simulink model "PMT_MPPT"  (Simulink 8.4)
settings: Solver=ode45  StartTime=0.0  StopTime=8  FixedStep=2.5e-6  RelTol=1e-3
undefined symbols (not defined in the file): Cin, Cout, Cp, G, Isc, L1a, L1b, Rload, Rload1, Rload2, sigbuilder_block, T1, T2, Temp, Tsampling, Voc
libraries: powerlib x19, simulink x3, powerlib_extras x1, fuzblock x1
settings Model: Creator=daoxuanb  LastModifiedBy=Administrator

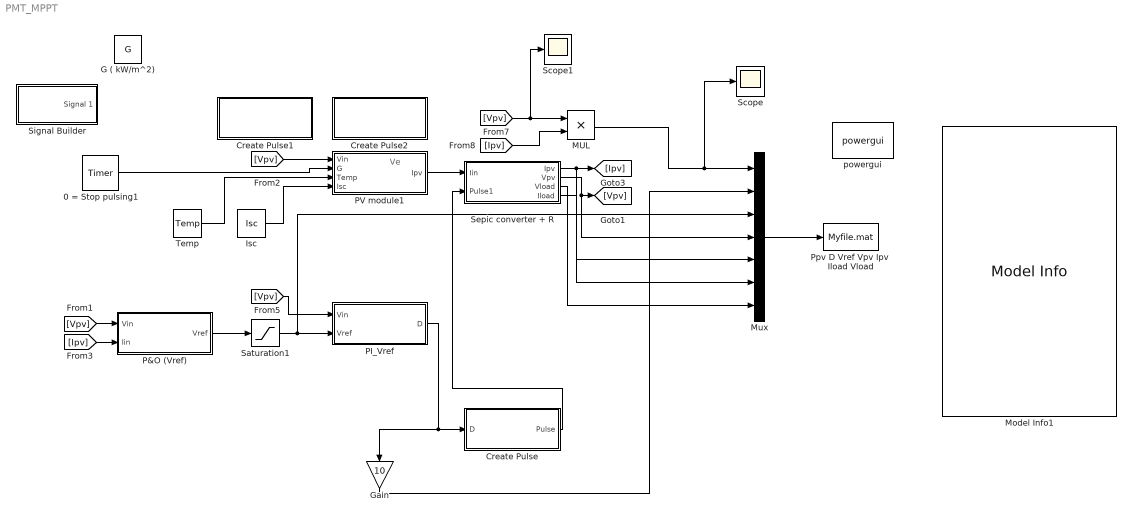
== system PMT_MPPT ==
  note: Ve
  0 = Stop pulsing1 : powerlib_extras/Control  Blocks/Timer  t=[0 2 4 6 8 ]  e=[1 0.9 0.8 0.6 0.5 ]
  Create Pulse : Subsystem
  Create Pulse1 : Subsystem
      settings: OpenFcn=thongso1
      mask Display: disp('initiate')
  Create Pulse2 : Subsystem
      settings: OpenFcn=ve1
      mask Display: disp('initiate')
  G ( kW/m^2) : Constant  Value=G
  Gain : Gain  Gain=10
  Isc : Constant  Value=Isc
  MUL : Product  Inputs=**
  Model Info1 : simulink/Model-Wide Utilities/Model Info  BlockCM=None  Frame=on  DisplayStringWithTags=|  HorizontalTextAlignment=Center  LeftAlignmentValue=0.5  SourceBlockDiagram=PMT_MPPT  TagMaxNumber=20
      | PARAMETER:
      | Boost + R:
      | C1 = 1000uF
      | C2 = 1000uF
      | C3 = 1000uF
      | L1 = 222uH
      | L2 = 222uH
      | R   = 20
      | Boost + Motor:
      | C1 = 2200u
      | C2 = 100u
      | L   = 10m
      | R   = 20
      | PI:  P = 0.05  I = 1
      | Pulse: 20000Hz
      | Pmax =  85W
      | Vmpp = 18.18 V
      | Impp   =  4.88 A
      | Voc = 21.85 V
      | Isc = 5.13 A
  Mux : Mux  Inputs=7
  P&O (Vref) : Subsystem
  PI_Vref : Subsystem
  PV module1 : Subsystem
  Ppv D Vref Vpv Ipv  Iload Vload : ToFile  Filename=Myfile.mat  MatrixName=XX
  Saturation1 : Saturate  UpperLimit=21.85  LowerLimit=0
  Scope : Scope
      settings: YMin=30  YMax=90  SaveName=Ppv
  Scope1 : Scope
      settings: YMin=10  YMax=90  SaveName=Ppv1
  Sepic converter + R : Subsystem
  Signal Builder : Subsystem  Tag=STV Subsys  LoadFcn=sigbuilder_block('load');  StartFcn=sigbuilder_block('start');  StopFcn=sigbuilder_block('stop');  ClipboardFcn=sigbuilder_block('clipboard');  mask(Sigbuilder block){}
      mask help: Simulink:masks:SigbuilderBlock_MD
      mask init:
      | if ~strcmp(get_param(bdroot(gcbh),'SimulationStatus'),'stopped') tuvar = sigbuilder_block('maskInit'); end
      settings: CopyFcn=sigbuilder_block('copy');  DeleteFcn=sigbuilder_block('delete');  ModelCloseFcn=sigbuilder_block('modelClose');  PreSaveFcn=sigbuilder_block('preSave');  PauseFcn=sigbuilder_block('pause');  ContinueFcn=sigbuilder_block('continue');  NameChangeFcn=sigbuilder_block('namechange');  OpenFcn=sigbuilder_block('open',[584.25 105.75 550.5 399.75 ]);  CloseFcn=sigbuilder_block('close');
      mask Display: plot(0, 0, 100, 100,[2, 2, 32, 32, 2], [68, 8, 8, 68, 68],[32, 2], [38, 38], [32, 19, 2],[53, 60, 44], [32, 17, 17, 2],[16, 16, 31, 31]);txt = getActiveGroup(gcbh);text(2, 100, txt,'verticalAlignment', 'top');
  "Temp " : Constant  Value=Temp
  powergui : powerlib/powergui  Priority=1  SimulationMode=Discrete  SolverType=Tustin  SampleTime=1e-5  frequency=60  SPID=off  DisableSnubberDevices=off  DisableRonSwitches=off  DisableVfSwitches=off  SwTol=0  DisplayEquations=off  Interpol=off  methode=off  Ts=0  frequencyindice=0  Pbase=100e6  ErrMax=1e-4  Iterations=50  UnitsV=kV  UnitsW=MW  FunctionMessages=off  echomessages=off  HookPort=off  EnableUseOfTLC=off  x0status=blocks  RestoreLinks=warning  ResistiveCurrentMeasurement=off  Frange=[0:2:500]  Ylog=off  Xlog=on  ShowGrid=off  save=off  variable=ZData  structure=0  ZoomFFT=off  StartTime=0.0  cycles=1  DisplayStyle=1  fundamental=60  FreqAxis=off  MaxFrequency=1000  frequencyindicesteady=1  RmsSteady=1  display=off
  wires:
  Saturation1/1 -> PI_Vref/2(Vref), Mux/3
  Create Pulse/1(Pulse) -> Sepic converter + R/2(Pulse1)
  [Vpv] -> P&O (Vref)/1(Vin)
  [Ipv] -> P&O (Vref)/2(Iin)
  Isc/1 -> PV module1/4(Isc)
  "Temp "/1 -> PV module1/3(Temp)
  [Vpv] -> PI_Vref/1(Vin)
  P&O (Vref)/1(Vref) -> Saturation1/1
  Sepic converter + R/1(Ipv) -> [Ipv], Mux/5
  Sepic converter + R/2(Vpv) -> Mux/4, [Vpv]
  PV module1/1(Ipv) -> Sepic converter + R/1(Iin)
  [Vpv] -> Scope1/1, MUL/1
  [Ipv] -> MUL/2
  MUL/1 -> Scope/1, Mux/1
  Gain/1 -> Mux/2
  Sepic converter + R/4(Iload) -> Mux/6
  Sepic converter + R/3(Vload) -> Mux/7
  Mux/1 -> Ppv D Vref Vpv Ipv  Iload Vload/1
  [Vpv] -> PV module1/1(Vin)
  PI_Vref/1(D) -> Gain/1, Create Pulse/1(D)
  0 = Stop pulsing1/1 -> PV module1/2(G)

== system PMT_MPPT/Create Pulse ==
  D : Inport
  Relay : Relay
  Repeating Sequence : simulink/Sources/Repeating Sequence  rep_seq_t=[0 1/1000]  rep_seq_y=[0 1]
  Sum : Sum  Inputs=|+-
  Pulse : Outport
  wires:
  D/1 -> Sum/1
  Repeating Sequence/1 -> Sum/2
  Sum/1 -> Relay/1
  Relay/1 -> Pulse/1

== system PMT_MPPT/Create Pulse1 ==

== system PMT_MPPT/Create Pulse2 ==

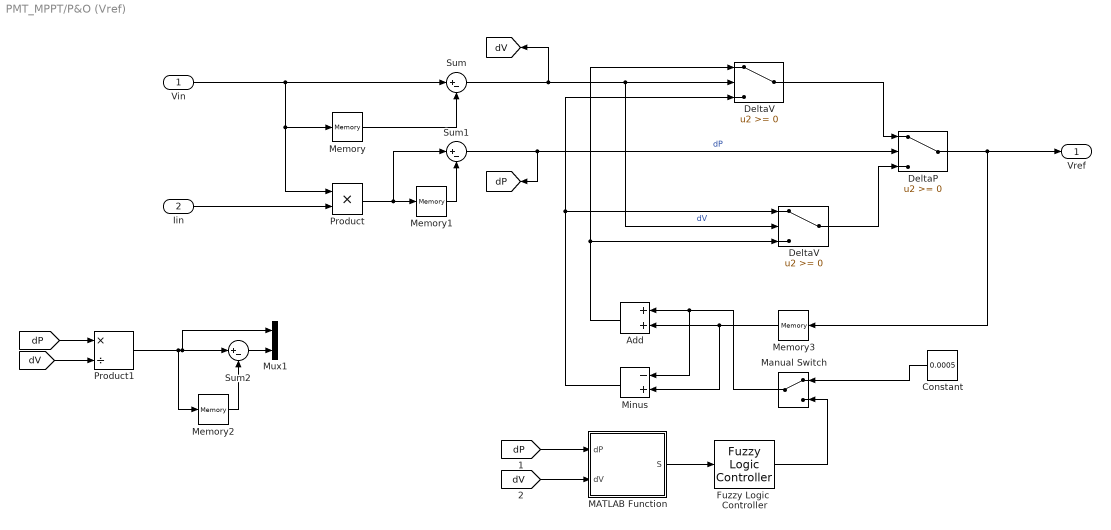
== system PMT_MPPT/P&O (Vref) ==
  Vin : Inport
  Iin : Inport  Port=2
  Add : Sum
  Constant : Constant  Value=0.0005  VectorParams1D=off
  DeltaP : Switch
  DeltaV : Switch
  "DeltaV " : Switch
  Fuzzy Logic  Controller : fuzblock/Fuzzy Logic  Controller  fis=['fuzzy1.fis']
  MATLAB Function : MATLAB Function  TreatAsAtomicUnit=on
  Manual Switch : ManualSwitch
  Memory : Memory  LinearizeMemory=on
  Memory1 : Memory
  Memory2 : Memory  LinearizeMemory=on
  Memory3 : Memory  X0=0.1
  Minus : Sum  Inputs=-+
  Mux1 : Mux  Inputs=2
  Product : Product
  Product1 : Product  Inputs=*/
  Sum : Sum  Inputs=|+-
  Sum1 : Sum  Inputs=|+-
  Sum2 : Sum  Inputs=|+-
  Vref : Outport
  tag scope: dP=global, dV=global
  wires:
  Memory/1 -> Sum/2
  Memory1/1 -> Sum1/2
  Vin/1 -> Sum/1, Memory/1, Product/1
  Iin/1 -> Product/2
  Product/1 -> Memory1/1, Sum1/1
  "DeltaV "/1 -> DeltaP/1
  DeltaV/1 -> DeltaP/3
  Sum1/1 -> DeltaP/2, [dP]  "dP"
  Sum/1 -> [dV], "DeltaV "/2, DeltaV/2  "dV"
  DeltaP/1 -> Memory3/1, Vref/1
  Memory3/1 -> Minus/2, Add/2
  Add/1 -> "DeltaV "/1, DeltaV/3
  Minus/1 -> "DeltaV "/3, DeltaV/1
  [dP] -> Product1/1
  [dV] -> Product1/2
  Product1/1 -> Sum2/1, Mux1/1, Memory2/1
  Memory2/1 -> Sum2/2
  Sum2/1 -> Mux1/2
  [dP] -> MATLAB Function/1(dP)
  [dV] -> MATLAB Function/2(dV)
  MATLAB Function/1(S) -> Fuzzy Logic  Controller/1
  Constant/1 -> Manual Switch/1
  Manual Switch/1 -> Minus/1, Add/1
  Fuzzy Logic  Controller/1 -> Manual Switch/2

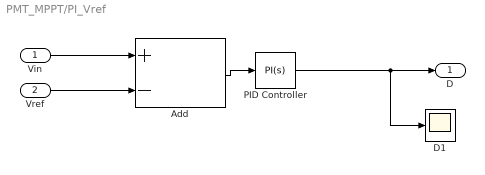
== system PMT_MPPT/PI_Vref ==
  Vin : Inport
  Vref : Inport  Port=2
  Add : Sum  Inputs=+-
  D1 : Scope
      settings: YMin=0.1  YMax=0.95  SaveName=ScopeData4
  PID Controller : simulink/Continuous/PID Controller  Controller=PI  TimeDomain=Continuous-time  SampleTime=-1  IntegratorMethod=Forward Euler  FilterMethod=Forward Euler  Form=Parallel  P=0.05  I=1  D=0  N=100  InitialConditionSource=internal  InitialConditionForIntegrator=0  InitialConditionForFilter=0  ExternalReset=none  LimitOutput=on  UpperSaturationLimit=0.95  LowerSaturationLimit=0  LinearizeAsGain=off  AntiWindupMode=back-calculation  Kb=1  TrackingMode=off  Kt=1  PParamMin=[]  PParamMax=[]  IParamMin=[]  IParamMax=[]  DParamMin=[]  DParamMax=[]  NParamMin=[]  NParamMax=[]  KbParamMin=[]  KbParamMax=[]  KtParamMin=[]  KtParamMax=[]  POutMin=[]  POutMax=[]  IOutMin=[]  IOutMax=[]  DOutMin=[]  DOutMax=[]  NOutMin=[]  NOutMax=[]  KbOutMin=[]  KbOutMax=[]  KtOutMin=[]  KtOutMax=[]  IntegratorOutMin=[]  IntegratorOutMax=[]  FilterOutMin=[]  FilterOutMax=[]  SumOutMin=[]  SumOutMax=[]  SumI1OutMin=[]  SumI1OutMax=[]  SumI2OutMin=[]  SumI2OutMax=[]  SumI3OutMin=[]  SumI3OutMax=[]  SumDOutMin=[]  SumDOutMax=[]  SaturationOutMin=[]  SaturationOutMax=[]  IntegratorContinuousStateAttributes=''  IntegratorStateMustResolveToSignalObject=off  IntegratorRTWStateStorageClass=Auto  FilterContinuousStateAttributes=''  FilterStateMustResolveToSignalObject=off  FilterRTWStateStorageClass=Auto  DifferentiatorICPrevScaledInput=0  DifferentiatorOutMin=[]  DifferentiatorOutMax=[]  UseFilter=on
  D : Outport
  wires:
  Vref/1 -> Add/2
  Vin/1 -> Add/1
  Add/1 -> PID Controller/1
  PID Controller/1 -> D/1, D1/1

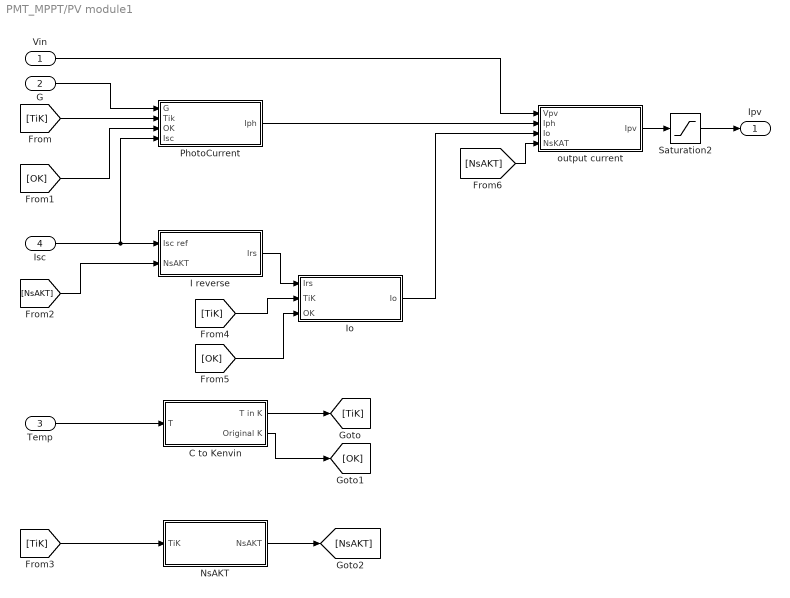
== system PMT_MPPT/PV module1 ==
  Vin : Inport
  G : Inport  Port=2
  Temp : Inport  Port=3
  Isc : Inport  Port=4
  C to Kenvin : Subsystem
  I reverse : Subsystem
  Io : Subsystem
  NsAKT : Subsystem
  PhotoCurrent : Subsystem
  Saturation2 : Saturate  UpperLimit=5.13  LowerLimit=0
  output current : Subsystem
  Ipv : Outport
  wires:
  Saturation2/1 -> Ipv/1
  [NsAKT] -> I reverse/2(NsAKT)
  PhotoCurrent/1(Iph) -> output current/2(Iph)
  [OK] -> PhotoCurrent/3(OK)
  [TiK] -> PhotoCurrent/2(Tik)
  G/1 -> PhotoCurrent/1(G)
  Io/1(Io) -> output current/3(Io)
  Vin/1 -> output current/1("Vpv ")
  Isc/1 -> PhotoCurrent/4(Isc), I reverse/1(Isc ref)
  [NsAKT] -> output current/4(NsKAT)
  NsAKT/1(NsAKT) -> [NsAKT]
  [TiK] -> NsAKT/1(TiK)
  output current/1(Ipv) -> Saturation2/1
  [OK] -> Io/3(OK)
  [TiK] -> Io/2(TiK)
  I reverse/1(Irs) -> Io/1(Irs)
  C to Kenvin/2(Original K) -> [OK]
  C to Kenvin/1(T in K) -> [TiK]
  Temp/1 -> C to Kenvin/1(T)

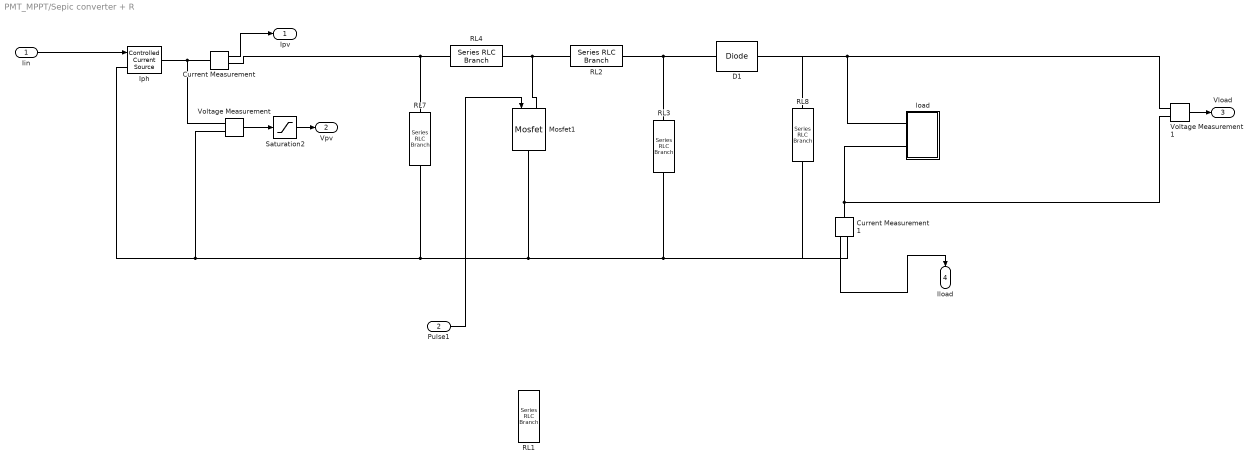
== system PMT_MPPT/Sepic converter + R ==
  Iin : Inport
  Pulse1 : Inport  Port=2
  Current Measurement : powerlib/Measurements/Current Measurement  PhasorSimulation=off  OutputType=Complex  PSBequivalent=0
  Current Measurement1 : powerlib/Measurements/Current Measurement  PhasorSimulation=off  OutputType=Complex  PSBequivalent=0
  D1 : powerlib/Power Electronics/Diode  Ron=0.001  Lon=0  Vf=0.8  IC=0  UseSnubber=off  Rs=500  Cs=250e-9  Measurements=off
  Iph : powerlib/Electrical Sources/Controlled Current Source  Initialize=on  Source_Type=DC  Amplitude=0  Phase=0  Frequency=0  Measurements=None
  Mosfet1 : powerlib/Power Electronics/Mosfet  Ron=0.1  Lon=0  Rd=0.01  Vfd=0  IC=0  Rs=1e5  Cs=inf  Measurements=off
  RL1 : powerlib/Elements/Series RLC Branch  LConnTagsString=__new0  RConnTagsString=__new0  BranchType=R  Resistance=Rload  Inductance=10e-3  SetiL0=off  InitialCurrent=0  Capacitance=1e-6  Setx0=off  InitialVoltage=0  Measurements=None
  RL2 : powerlib/Elements/Series RLC Branch  LConnTagsString=__new0  RConnTagsString=__new0  BranchType=C  Resistance=20  Inductance=1e-3  SetiL0=off  InitialCurrent=0  Capacitance=Cp  Setx0=off  InitialVoltage=0  Measurements=None
  RL3 : powerlib/Elements/Series RLC Branch  LConnTagsString=__new0  RConnTagsString=__new0  BranchType=L  Resistance=10  Inductance=L1b  SetiL0=off  InitialCurrent=0  Capacitance=1e-6  Setx0=off  InitialVoltage=0  Measurements=None
  RL4 : powerlib/Elements/Series RLC Branch  LConnTagsString=__new0  RConnTagsString=__new0  BranchType=L  Resistance=10  Inductance=L1a  SetiL0=off  InitialCurrent=0  Capacitance=1e-6  Setx0=off  InitialVoltage=0  Measurements=None
  RL7 : powerlib/Elements/Series RLC Branch  LConnTagsString=__new0  RConnTagsString=__new0  BranchType=C  Resistance=20  Inductance=1e-3  SetiL0=off  InitialCurrent=0  Capacitance=Cin  Setx0=off  InitialVoltage=0  Measurements=None
  RL8 : powerlib/Elements/Series RLC Branch  LConnTagsString=__new0  RConnTagsString=__new0  BranchType=C  Resistance=20  Inductance=1e-3  SetiL0=off  InitialCurrent=0  Capacitance=Cout  Setx0=off  InitialVoltage=0  Measurements=None
  Saturation2 : Saturate  UpperLimit=21.85  LowerLimit=0
  Voltage Measurement : powerlib/Measurements/Voltage Measurement  PhasorSimulation=off  OutputType=Complex  PSBequivalent=0
  Voltage Measurement1 : powerlib/Measurements/Voltage Measurement  PhasorSimulation=off  OutputType=Complex  PSBequivalent=0
  load : Subsystem
  Ipv : Outport
  Vpv : Outport  Port=2
  Vload : Outport  Port=3
  Iload : Outport  Port=4
  wires:
  Voltage Measurement/1 -> Saturation2/1
  Current Measurement/1 -> Ipv/1
  Iin/1 -> Iph/1
  Saturation2/1 -> Vpv/1
  Current Measurement1/1 -> Iload/1
  Voltage Measurement1/1 -> Vload/1
  Pulse1/1 -> Mosfet1/1
  connections:
  Current Measurement/LConn1 -- Iph/RConn1 -- Voltage Measurement/LConn1
  RL8/LConn1 -- D1/RConn1 -- load/LConn1 -- Voltage Measurement1/LConn1
  Current Measurement1/LConn1 -- load/LConn2 -- Voltage Measurement1/LConn2
  RL7/LConn1 -- Current Measurement/RConn1 -- RL4/RConn1
  RL4/LConn1 -- RL2/LConn1 -- Mosfet1/LConn1
  RL3/RConn1 -- RL8/RConn1 -- Current Measurement1/RConn1 -- Mosfet1/RConn1 -- Iph/LConn1 -- Voltage Measurement/LConn2 -- RL7/RConn1
  RL2/RConn1 -- RL3/LConn1 -- D1/LConn1

== system PMT_MPPT/Signal Builder ==
  Demux : Demux  Tag=STV Demux  Outputs=1
  FromWs : FromWorkspace  Tag=STV FromWs  VariableName=tuvar  SampleTime=0  SigBuilderData=DataTag0  VnvData=DataTag1
      SigBuilderData=|
      | common.afterFinalStr = 'Extrapolate'
      | common.sampleTime = 0
      | dataSet.timeRange = [0 10]
      | dataSet.name = 'Group 1'
      | sbobj.Groups.Name = 'Group 1'
      | sbobj.Groups.Signals.Name = 'Signal 1'
      | sbobj.Groups.Signals.XData = [0 2.98 2.98 5 5 10]
      | sbobj.Groups.Signals.YData = [1 1 0.5 0.5 0.8 0.8]
  Signal 1 : Outport  Tag=STV Outport
  wires:
  Demux/1 -> Signal 1/1
  FromWs/1 -> Demux/1

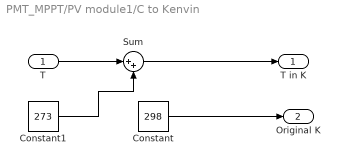
== system PMT_MPPT/PV module1/C to Kenvin ==
  T : Inport
  Constant : Constant  Value=298
  Constant1 : Constant  Value=273
  Sum : Sum  Inputs=|++
  T in K : Outport
  Original K : Outport  Port=2
  wires:
  Sum/1 -> T in K/1
  Constant1/1 -> Sum/2
  T/1 -> Sum/1
  Constant/1 -> Original K/1

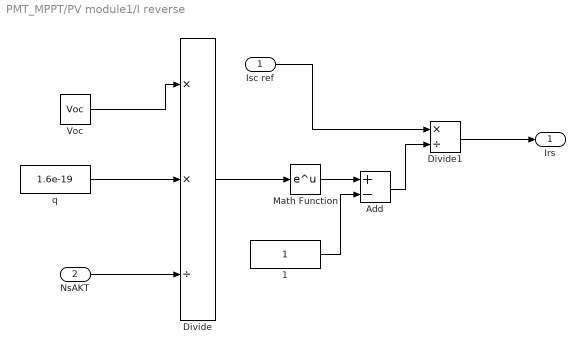
== system PMT_MPPT/PV module1/I reverse ==
  Isc ref : Inport
  NsAKT : Inport  Port=2
  1 : Constant
  Add : Sum  Inputs=+-
  Divide : Product  Inputs=**/
  Divide1 : Product  Inputs=*/
  Math Function : Math  SaturateOnIntegerOverflow=on
  Voc : Constant  Value=Voc
  q : Constant  Value=1.6e-19
  Irs : Outport
  wires:
  Add/1 -> Divide1/2
  1/1 -> Add/2
  Math Function/1 -> Add/1
  q/1 -> Divide/2
  NsAKT/1 -> Divide/3
  Voc/1 -> Divide/1
  Divide1/1 -> Irs/1
  Divide/1 -> Math Function/1
  Isc ref/1 -> Divide1/1

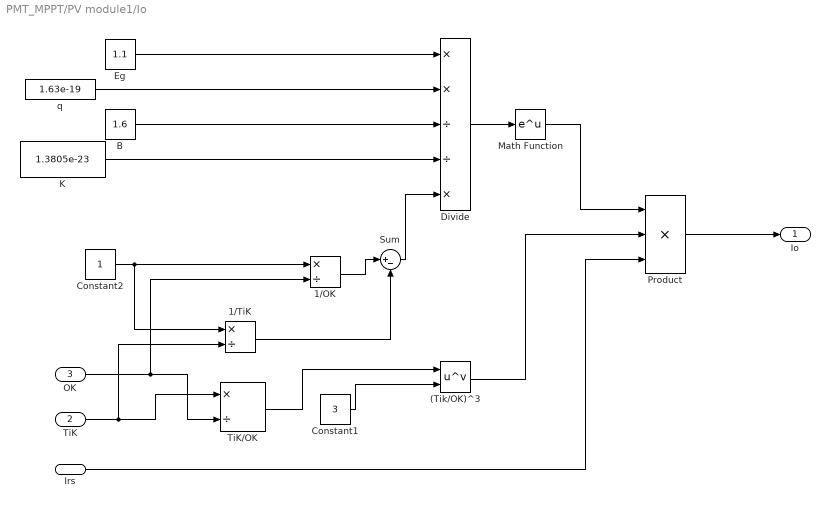
== system PMT_MPPT/PV module1/Io ==
  Irs : Inport
  TiK : Inport  Port=2
  OK : Inport  Port=3
  (Tik/OK)^3 : Math  Operator=pow  SaturateOnIntegerOverflow=on
  1/OK : Product  Inputs=*/
  1/TiK : Product  Inputs=*/
  B : Constant  Value=1.6
  Constant1 : Constant  Value=3
  Constant2 : Constant
  Divide : Product  Inputs=**//*
  Eg : Constant  Value=1.1
  K : Constant  Value=1.3805e-23
  Math Function : Math  SaturateOnIntegerOverflow=on
  Product : Product  Inputs=3  RndMeth=Zero
  Sum : Sum  Inputs=|+-
  TiK/OK : Product  Inputs=*/
  q : Constant  Value=1.63e-19
  Io : Outport
  wires:
  Constant1/1 -> (Tik/OK)^3/2
  Irs/1 -> Product/3
  (Tik/OK)^3/1 -> Product/2
  Sum/1 -> Divide/5
  1/TiK/1 -> Sum/2
  1/OK/1 -> Sum/1
  Constant2/1 -> 1/OK/1, 1/TiK/1
  Product/1 -> Io/1
  Math Function/1 -> Product/1
  Divide/1 -> Math Function/1
  K/1 -> Divide/4
  B/1 -> Divide/3
  q/1 -> Divide/2
  Eg/1 -> Divide/1
  TiK/OK/1 -> (Tik/OK)^3/1
  OK/1 -> TiK/OK/2, 1/OK/2
  TiK/1 -> TiK/OK/1, 1/TiK/2

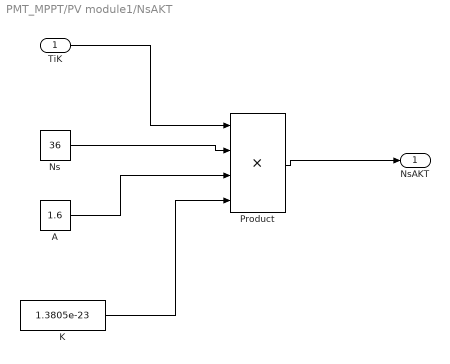
== system PMT_MPPT/PV module1/NsAKT ==
  TiK : Inport
  A : Constant  Value=1.6
  K : Constant  Value=1.3805e-23
  Ns : Constant  Value=36
  Product : Product  Inputs=4  RndMeth=Zero
  NsAKT : Outport
  wires:
  K/1 -> Product/4
  A/1 -> Product/3
  Product/1 -> NsAKT/1
  Ns/1 -> Product/2
  TiK/1 -> Product/1

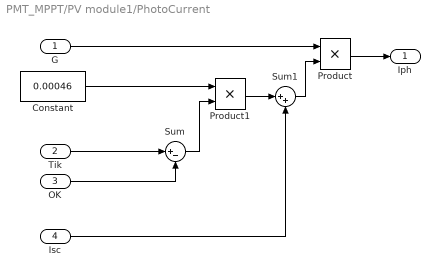
== system PMT_MPPT/PV module1/PhotoCurrent ==
  G : Inport
  Tik : Inport  Port=2
  OK : Inport  Port=3
  Isc : Inport  Port=4
  Constant : Constant  Value=0.00046
  Product : Product  RndMeth=Zero
  Product1 : Product  RndMeth=Zero
  Sum : Sum  Inputs=|+-
  Sum1 : Sum  Inputs=|++
  Iph : Outport
  wires:
  Product/1 -> Iph/1
  Sum1/1 -> Product/2
  Product1/1 -> Sum1/1
  Isc/1 -> Sum1/2
  G/1 -> Product/1
  Constant/1 -> Product1/1
  Sum/1 -> Product1/2
  OK/1 -> Sum/2
  Tik/1 -> Sum/1

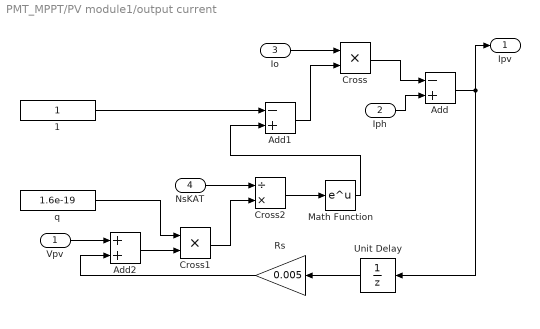
== system PMT_MPPT/PV module1/output current ==
  "Vpv " : Inport
  Iph : Inport  Port=2
  Io : Inport  Port=3
  NsKAT : Inport  Port=4
  1 : Constant
  Add : Sum  Inputs=-+
  Add1 : Sum  Inputs=-+
  Add2 : Sum
  Cross : Product  Inputs=**
  Cross1 : Product  Inputs=**
  Cross2 : Product  Inputs=/*
  Math Function : Math  SaturateOnIntegerOverflow=on
  Rs : Gain  Gain=0.005
  Unit Delay : UnitDelay  SampleTime=-1
  q : Constant  Value=1.6e-19
  Ipv : Outport
  wires:
  Math Function/1 -> Add1/2
  Cross2/1 -> Math Function/1
  NsKAT/1 -> Cross2/1
  Cross1/1 -> Cross2/2
  q/1 -> Cross1/1
  Add2/1 -> Cross1/2
  Rs/1 -> Add2/2
  "Vpv "/1 -> Add2/1
  Unit Delay/1 -> Rs/1
  1/1 -> Add1/1
  Add1/1 -> Cross/2
  Io/1 -> Cross/1
  Cross/1 -> Add/1
  Add/1 -> Unit Delay/1, Ipv/1
  Iph/1 -> Add/2

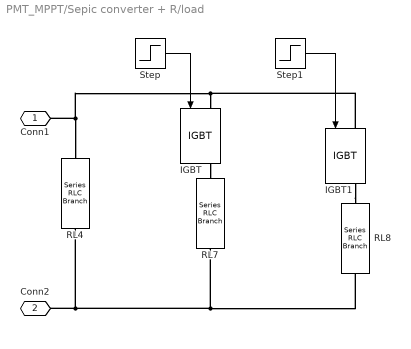
== system PMT_MPPT/Sepic converter + R/load ==
  IGBT : powerlib/Power Electronics/IGBT  Ron=0.001  Lon=0  Vf=1  Tf=1e-6  Tt=2e-6  IC=0  Rs=1e5  Cs=inf  Measurements=on
  IGBT1 : powerlib/Power Electronics/IGBT  Ron=0.001  Lon=0  Vf=1  Tf=1e-6  Tt=2e-6  IC=0  Rs=1e5  Cs=inf  Measurements=on
  RL4 : powerlib/Elements/Series RLC Branch  LConnTagsString=__new0  RConnTagsString=__new0  BranchType=R  Resistance=Rload  Inductance=10e-3  SetiL0=off  InitialCurrent=0  Capacitance=1e-6  Setx0=off  InitialVoltage=0  Measurements=None
  RL7 : powerlib/Elements/Series RLC Branch  LConnTagsString=__new0  RConnTagsString=__new0  BranchType=R  Resistance=Rload1  Inductance=10e-3  SetiL0=off  InitialCurrent=0  Capacitance=1e-6  Setx0=off  InitialVoltage=0  Measurements=None
  RL8 : powerlib/Elements/Series RLC Branch  LConnTagsString=__new0  RConnTagsString=__new0  BranchType=R  Resistance=Rload2  Inductance=10e-3  SetiL0=off  InitialCurrent=0  Capacitance=1e-6  Setx0=off  InitialVoltage=0  Measurements=None
  Step : Step  Time=T1  SampleTime=Tsampling
  Step1 : Step  Time=T2  SampleTime=Tsampling
  Conn1 : PMIOPort  Port=1  Side=Left
  Conn2 : PMIOPort  Port=2  Side=Left
  wires:
  Step/1 -> IGBT/1
  Step1/1 -> IGBT1/1
  connections:
  IGBT1/LConn1 -- Conn1/RConn1 -- RL4/RConn1 -- IGBT/LConn1
  IGBT/RConn1 -- RL7/RConn1
  IGBT1/RConn1 -- RL8/LConn1
  RL8/RConn1 -- RL7/LConn1 -- RL4/LConn1 -- Conn2/RConn1

== matlab function P&O (Vref)/MATLAB Function ==
  data: dP input double; S output double; dV input double
function S = fcn(dP,dV)
%#codegen

S=abs(dP/dV);
